simulink model "GNC"  (R2015b)
settings: Solver=ode45  StartTime=0.0  StopTime=15  MaxStep=0.1  RelTol=1e-3
InitFcn:
  | % load parameters of the default quadrotor
  | disp('Quadrotor parameters loaded by InitFcn')
  | mdl_quadrotor
undefined symbols (not defined in the file or in its folder): quad
libraries: roblocks x1, simulink x1
settings Model: Creator=corkep  LastModifiedBy=Borja
settings DataIOCC: SaveFormat=Array  SignalLoggingSaveFormat=ModelDataLogs
settings OptimizationCC: ExpressionDepthLimit=2147483647
settings DebuggingCC: UnderspecifiedInitializationDetection=Classic  MergeDetectMultiDrivingBlocksExec=none  SolverPrmCheckMsg=warning  FcnCallInpInsideContextMsg=UseLocalSettings  StateNameClashWarn=warning
settings HardwareCC: ProdBitPerPointer=32  ProdLargestAtomicFloat=None  ProdIntDivRoundTo=Undefined  ProdEndianess=Unspecified  ProdWordSize=32  ProdHWDeviceType=32-bit Generic
settings GRTTargetCC: GeneratePreprocessorConditionals=Disable all  CombineOutputUpdateFcns=off  GRTInterface=on
settings ConfigComp: CovModelRefEnable=Off  CovSFcnEnable=off

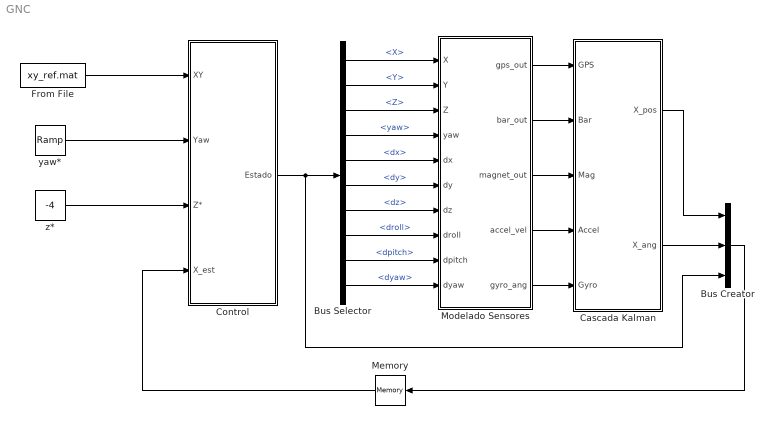
== system GNC ==
  Bus Creator : BusCreator  Inputs=3
  Bus Selector : BusSelector  OutputSignals=X,Y,Z,yaw,dx,dy,dz,droll,dpitch,dyaw
  Cascada Kalman : Subsystem
  Control : Subsystem
  From File : FromFile  FileName=xy_ref.mat  SampleTime=0
  Memory : Memory  InheritSampleTime=on
  Modelado Sensores : Subsystem
  yaw* : simulink/Sources/Ramp  slope=0.2  start=2  X0=0
  z* : Constant  Value=-4  SampleTime=0
  wires:
  Bus Selector/1 -> Modelado Sensores/1(X)  "<X>"
  Bus Selector/2 -> Modelado Sensores/2(Y)  "<Y>"
  Bus Selector/3 -> Modelado Sensores/3(Z)  "<Z>"
  Bus Selector/4 -> Modelado Sensores/4(yaw)  "<yaw>"
  Bus Selector/5 -> Modelado Sensores/5(dx)  "<dx>"
  Bus Selector/6 -> Modelado Sensores/6(dy)  "<dy>"
  Bus Selector/7 -> Modelado Sensores/7(dz)  "<dz>"
  Bus Selector/10 -> Modelado Sensores/10(dyaw)  "<dyaw>"
  Bus Selector/9 -> Modelado Sensores/9(dpitch)  "<dpitch>"
  Bus Selector/8 -> Modelado Sensores/8(droll)  "<droll>"
  Modelado Sensores/2(bar_out) -> Cascada Kalman/2(Bar)
  Modelado Sensores/3(magnet_out) -> Cascada Kalman/3(Mag)
  Modelado Sensores/4(accel_vel) -> Cascada Kalman/4(Accel)
  Modelado Sensores/5(gyro_ang) -> Cascada Kalman/5(Gyro)
  Control/1(Estado) -> Bus Creator/3, Bus Selector/1
  Cascada Kalman/1(X_pos) -> Bus Creator/1
  Bus Creator/1 -> Memory/1
  Cascada Kalman/2(X_ang) -> Bus Creator/2
  z*/1 -> Control/3(Z*)
  yaw*/1 -> Control/2(Yaw)
  Memory/1 -> Control/4(X_est)
  Modelado Sensores/1(gps_out) -> Cascada Kalman/1(GPS)
  From File/1 -> Control/1(XY)

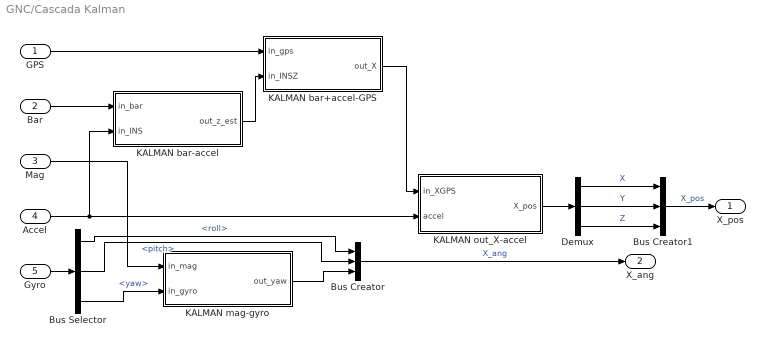
== system GNC/Cascada Kalman ==
  GPS : Inport
  Bar : Inport  Port=2
  Mag : Inport  Port=3
  Accel : Inport  Port=4
  Gyro : Inport  Port=5
  Bus Creator : BusCreator  Inputs=3
  Bus Creator1 : BusCreator  Inputs=3
  Bus Selector : BusSelector  OutputSignals=roll,pitch,yaw
  Demux : Demux  Outputs=3
  KALMAN bar+accel-GPS : Subsystem
  KALMAN bar-accel : Subsystem
  KALMAN mag-gyro : Subsystem
  KALMAN out_X-accel : Subsystem
  X_pos : Outport
  X_ang : Outport  Port=2
  wires:
  Accel/1 -> KALMAN out_X-accel/2(accel), KALMAN bar-accel/2(in_INS)
  GPS/1 -> KALMAN bar+accel-GPS/1(in_gps)
  KALMAN bar-accel/1(out_z_est) -> KALMAN bar+accel-GPS/2(in_INSZ)
  Bar/1 -> KALMAN bar-accel/1(in_bar)
  KALMAN bar+accel-GPS/1(out_X) -> KALMAN out_X-accel/1(in_XGPS)
  Gyro/1 -> Bus Selector/1
  Mag/1 -> KALMAN mag-gyro/1(in_mag)
  KALMAN mag-gyro/1(out_yaw) -> Bus Creator/3
  Bus Selector/2 -> Bus Creator/2  "<pitch>"
  Bus Selector/1 -> Bus Creator/1  "<roll>"
  Bus Selector/3 -> KALMAN mag-gyro/2(in_gyro)  "<yaw>"
  Bus Creator/1 -> X_ang/1  "X_ang"
  KALMAN out_X-accel/1(X_pos) -> Demux/1
  Demux/1 -> Bus Creator1/1  "X"
  Demux/2 -> Bus Creator1/2  "Y"
  Demux/3 -> Bus Creator1/3  "Z"
  Bus Creator1/1 -> X_pos/1  "X_pos"

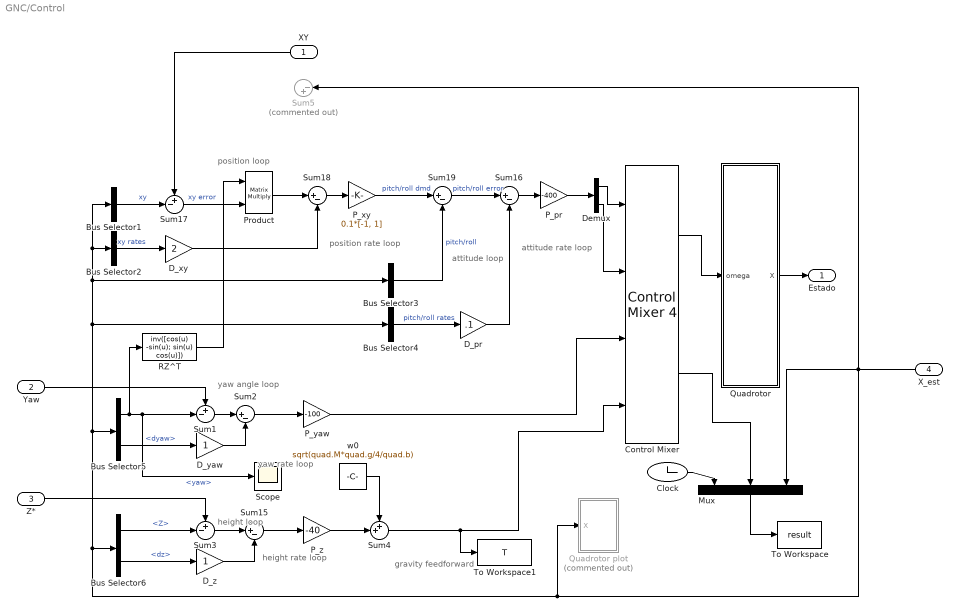
== system GNC/Control ==
  note: gravity feedforward
  note: attitude rate
      | loop
  note: attitude
      | loop
  note: position rate
      | loop
  note: position
      | loop
  note: yaw rate
      | loop
  note: yaw angle
      | loop
  note: height rate
      | loop
  note: height
      | loop
  XY : Inport
  Yaw : Inport  Port=2
  Z* : Inport  Port=3
  X_est : Inport  Port=4
  Bus Selector1 : BusSelector  OutputSignals=X_pos.X,X_pos.Y  OutputAsBus=on
  Bus Selector2 : BusSelector  OutputSignals=signal3.dx,signal3.dy  OutputAsBus=on
  Bus Selector3 : BusSelector  OutputSignals=X_ang.pitch,X_ang.roll  OutputAsBus=on
  Bus Selector4 : BusSelector  OutputSignals=signal3.dpitch,signal3.droll  OutputAsBus=on
  Bus Selector5 : BusSelector  OutputSignals=X_ang.yaw,signal3.dyaw
  Bus Selector6 : BusSelector  OutputSignals=X_pos.Z,signal3.dz
  Clock : Clock
  Control Mixer : roblocks/Dynamics/Control Mixer 4
  D_pr : Gain  Gain=.1
  D_xy : Gain  Gain=2
  D_yaw : Gain
  D_z : Gain
  Demux : Demux  Outputs=2
  Mux : Mux  Inputs=3
  P_pr : Gain  Gain=-400
  P_xy : Gain  Gain=0.1*[-1, 1]
  P_yaw : Gain  Gain=-100
  P_z : Gain  Gain=-40
  Product : Product  Multiplication=Matrix(*)  RndMeth=Zero
  Quadrotor : Subsystem  mask{quad=quad}
      mask prompts: quad "Quadrotor params"
      mask help: Quadrotor dynamics
      mask Help:
      | Integrate spatial velocity to update pose represented as a homogeneous
      | transformation.
      | 
      | <b>Parameters::</b>
      | 
      | q (struct)  A structure containing quadrotor dynamics
      | 
      | The elements of q are:
      | 
      |  J         Flyer rotational inertia matrix (3x3)
      |  h         Height of rotors above CoG (1x1)
      |  d         Length of flyer arms (1x1)
      |  nb        Number of blades per rotor (1x1)
      |  r         Rotor radius (1x1)
      |  c         Blade chord (1x1)
      |  e         Flapping hinge offset (1x1)
      |  Mb        Rotor blade mass (1x1)
      |  Mc        Estimated hub clamp mass (1x1)
      |  ec        Blade root clamp displacement (1x1)
      |  Ib        Rotor blade rotational inertia (1x1)
      |  Ic        Estimated root clamp inertia (1x1)
      |  mb        Static blade moment (1x1)
      |  Ir        Total rotor inertia (1x1)
      |  Ct        Non-dim. thrust coefficient (1x1)
      |  Cq        Non-dim. torque coefficient (1x1)
      |  sigma     Rotor solidity ratio (1x1)
      |  thetat    Blade tip angle (1x1)
      |  theta0    Blade root angle (1x1)
      |  theta1    Blade twist angle (1x1)
      |  theta75   3/4 blade angle (1x1)
      |  thetai    Blade ideal root approximation (1x1)
      |  a         Lift slope gradient (1x1)
      |  A         Rotor disc area (1x1)
      |  gamma     Lock number (1x1)
      | 
      | 
      | <b>Inputs::</b>
      | 
      | w1 (1x1) angular velocity of rotor 1 [rad]
      | w2 (1x1) angular velocity of rotor 2 [rad]
      | w3 (1x1) angular velocity of rotor 3 [rad]
      | w4 (1x1) angular velocity of rotor 4 [rad]
      | 
      | <b>Outputs::</b>
      | 
      | X (1x12) state vector (x, y, z, thr, thp, thy, xd, yd, zd, thrd, thpd, thyd)
      | 
      | (x,y,z) is the position in the world frame [m]
      | (thr, thp, thy) the roll/pitch/yaw orientation in the world frame [rad]
      | (xd,yd,zd) is the velocity in the body frame [m]
      | (thrd,thpd,thyd) is the roll/pitch/yaw rates in the body frame [rad/s]
      | 
      | <b>Notes::</b>
      | 
      | - See also mdl_quadrotor which defines parameters for the ANU X4 flyer.
  Quadrotor plot : Subsystem  Commented=on  mask{quad=quad, xydim=2, zdim=10}
      mask prompts: quad "Model"; xydim "xy-axes dimension"; zdim "z-axis dimension"
      mask help: Animate quadrotor.
      mask Help:
      | This block graphically displays a quadrotor (flying robot).
      | 
      | A new figure is created and A graphical model of a quadrotor is animated
      | to a pose specified by the state vector input to the block.
      | 
      | The state vector is [x y z roll pitch yaw] in world coordinates and the
      | angles are in radians.
      | 
      | Notes:
      | - The dimensions of the vehicle workspace are set by parameters
  RZ^T : MATLABFcn  MATLABFcn=inv([cos(u) -sin(u); sin(u) cos(u)])  OutputDimensions=[2 2]  Output1D=off
  Scope : Scope
  Sum1 : Sum  Inputs=+-|
  Sum{2,15..16,18..19} (5 alike) : Sum  Inputs=|+-
  Sum17 : Sum  Inputs=+-|
  Sum3 : Sum  Inputs=+-|
  Sum4 : Sum  Inputs=++|
  Sum5 : Sum  Commented=on  Inputs=|-+
  To Workspace : ToWorkspace  VariableName=result  SampleTime=-1
  To Workspace1 : ToWorkspace  VariableName=T  SampleTime=-1
  w0 : Constant  Value=sqrt(quad.M*quad.g/4/quad.b)  SampleTime=0
  Estado : Outport
  wires:
  w0/1 -> Sum4/1
  Sum15/1 -> P_z/1
  P_z/1 -> Sum4/2
  Quadrotor/1(X) -> Estado/1
  Bus Selector1/1 -> Sum17/2  "xy"
  Bus Selector2/1 -> D_xy/1  "xy rates"
  D_xy/1 -> Sum18/2
  P_xy/1 -> Sum19/1  "pitch/roll dmd"
  Bus Selector3/1 -> Sum19/2  "pitch/roll"
  Bus Selector4/1 -> D_pr/1  "pitch/roll rates"
  Sum19/1 -> Sum16/1  "pitch/roll error"
  Sum16/1 -> P_pr/1
  P_pr/1 -> Demux/1
  P_yaw/1 -> Control Mixer/3
  Bus Selector5/1 -> RZ^T/1, Sum1/2, Scope/1  "<yaw>"
  Sum2/1 -> P_yaw/1
  Z*/1 -> Sum3/1
  Bus Selector6/1 -> Sum3/2  "<Z>"
  Bus Selector5/2 -> D_yaw/1  "<dyaw>"
  Sum3/1 -> Sum15/1
  D_z/1 -> Sum15/2
  Bus Selector6/2 -> D_z/1  "<dz>"
  D_pr/1 -> Sum16/2
  Demux/2 -> Control Mixer/2
  D_yaw/1 -> Sum2/2
  Sum4/1 -> To Workspace1/1, Control Mixer/4
  Sum1/1 -> Sum2/1
  Mux/1 -> To Workspace/1
  Clock/1 -> Mux/1
  RZ^T/1 -> Product/1
  Sum18/1 -> P_xy/1
  Yaw/1 -> Sum1/1
  Product/1 -> Sum18/1
  Sum17/1 -> Product/2  "xy error"
  Demux/1 -> Control Mixer/1
  Control Mixer/1 -> Quadrotor/1(omega)
  X_est/1 -> Quadrotor plot/1(X), Bus Selector6/1, Bus Selector5/1, Bus Selector4/1, Bus Selector3/1, Bus Selector2/1, Bus Selector1/1, Sum5/1, Mux/3
  Control Mixer/2 -> Mux/2
  XY/1 -> Sum17/1

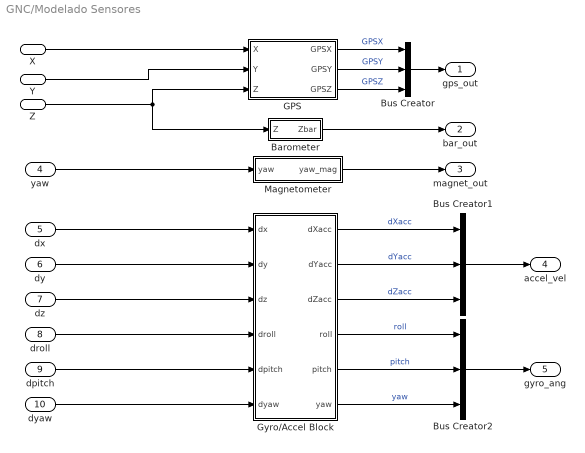
== system GNC/Modelado Sensores ==
  X : Inport
  Y : Inport  Port=2
  Z : Inport  Port=3
  yaw : Inport  Port=4
  dx : Inport  Port=5
  dy : Inport  Port=6
  dz : Inport  Port=7
  droll : Inport  Port=8
  dpitch : Inport  Port=9
  dyaw : Inport  Port=10
  Barometer : Subsystem
  Bus Creator : BusCreator  Inputs=3
  Bus Creator1 : BusCreator  Inputs='dXacc','dYacc','dZacc'
  Bus Creator2 : BusCreator  Inputs=3
  GPS : Subsystem
  Gyro/Accel Block : Subsystem
  Magnetometer : Subsystem
  gps_out : Outport
  bar_out : Outport  Port=2
  magnet_out : Outport  Port=3
  accel_vel : Outport  Port=4
  gyro_ang : Outport  Port=5
  wires:
  Bus Creator1/1 -> accel_vel/1
  Magnetometer/1(yaw_mag) -> magnet_out/1
  Bus Creator2/1 -> gyro_ang/1
  Barometer/1(Zbar) -> bar_out/1
  X/1 -> GPS/1(X)
  Y/1 -> GPS/2(Y)
  Z/1 -> GPS/3(Z), Barometer/1(Z)
  yaw/1 -> Magnetometer/1(yaw)
  GPS/1(GPSX) -> Bus Creator/1  "GPSX"
  GPS/2(GPSY) -> Bus Creator/2  "GPSY"
  GPS/3(GPSZ) -> Bus Creator/3  "GPSZ"
  Gyro/Accel Block/5(pitch) -> Bus Creator2/2  "pitch"
  Gyro/Accel Block/2(dYacc) -> Bus Creator1/2  "dYacc"
  Bus Creator/1 -> gps_out/1
  Gyro/Accel Block/1(dXacc) -> Bus Creator1/1  "dXacc"
  Gyro/Accel Block/3(dZacc) -> Bus Creator1/3  "dZacc"
  Gyro/Accel Block/6(yaw) -> Bus Creator2/3  "yaw"
  Gyro/Accel Block/4(roll) -> Bus Creator2/1  "roll"
  dx/1 -> Gyro/Accel Block/1(dx)
  dy/1 -> Gyro/Accel Block/2(dy)
  dz/1 -> Gyro/Accel Block/3(dz)
  dpitch/1 -> Gyro/Accel Block/5(dpitch)
  droll/1 -> Gyro/Accel Block/4(droll)
  dyaw/1 -> Gyro/Accel Block/6(dyaw)

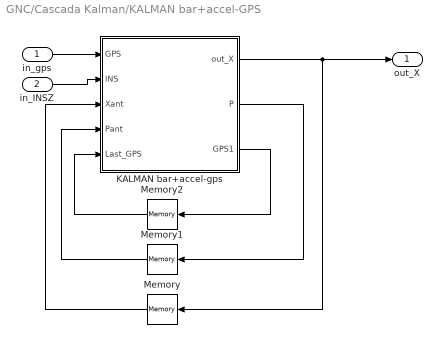
== system GNC/Cascada Kalman/KALMAN bar+accel-GPS ==
  in_gps : Inport
  in_INSZ : Inport  Port=2
  KALMAN bar+accel-gps : MATLAB Function  TreatAsAtomicUnit=on
  Memory : Memory  X0=[0;0;0]  InheritSampleTime=on
  Memory1 : Memory  X0=0.001  InheritSampleTime=on
  Memory2 : Memory  X0=0.001*[1;1;1]  InheritSampleTime=on
  out_X : Outport
  wires:
  in_gps/1 -> KALMAN bar+accel-gps/1(GPS)
  Memory/1 -> KALMAN bar+accel-gps/3(Xant)
  Memory1/1 -> KALMAN bar+accel-gps/4(Pant)
  KALMAN bar+accel-gps/3(GPS1) -> Memory2/1
  in_INSZ/1 -> KALMAN bar+accel-gps/2(INS)
  KALMAN bar+accel-gps/1(out_X) -> out_X/1, Memory/1
  KALMAN bar+accel-gps/2(P) -> Memory1/1
  Memory2/1 -> KALMAN bar+accel-gps/5(Last_GPS)

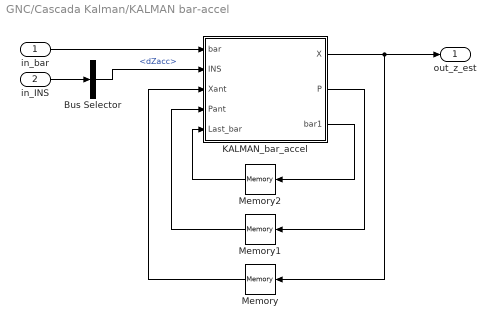
== system GNC/Cascada Kalman/KALMAN bar-accel ==
  in_bar : Inport
  in_INS : Inport  Port=2
  Bus Selector : BusSelector  OutputSignals=dZacc
  KALMAN_bar_accel : MATLAB Function  TreatAsAtomicUnit=on
  Memory : Memory
  Memory1 : Memory  X0=0.01  InheritSampleTime=on
  Memory2 : Memory  X0=0.001  InheritSampleTime=on
  out_z_est : Outport
  wires:
  in_bar/1 -> KALMAN_bar_accel/1(bar)
  KALMAN_bar_accel/1(X) -> Memory/1, out_z_est/1
  KALMAN_bar_accel/2(P) -> Memory1/1
  Memory1/1 -> KALMAN_bar_accel/4(Pant)
  Memory/1 -> KALMAN_bar_accel/3(Xant)
  KALMAN_bar_accel/3(bar1) -> Memory2/1
  Memory2/1 -> KALMAN_bar_accel/5(Last_bar)
  in_INS/1 -> Bus Selector/1
  Bus Selector/1 -> KALMAN_bar_accel/2(INS)  "<dZacc>"

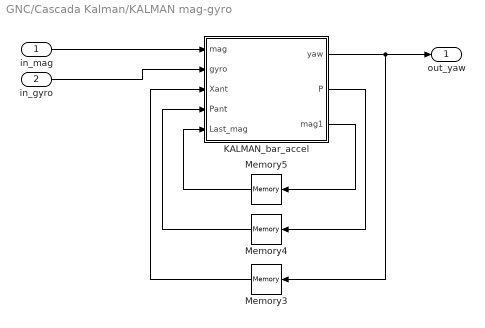
== system GNC/Cascada Kalman/KALMAN mag-gyro ==
  in_mag : Inport
  in_gyro : Inport  Port=2
  KALMAN_bar_accel : MATLAB Function  TreatAsAtomicUnit=on
  Memory3 : Memory  InheritSampleTime=on
  Memory4 : Memory  X0=0.01  InheritSampleTime=on
  Memory5 : Memory  X0=0.001  InheritSampleTime=on
  out_yaw : Outport
  wires:
  in_mag/1 -> KALMAN_bar_accel/1(mag)
  in_gyro/1 -> KALMAN_bar_accel/2(gyro)
  KALMAN_bar_accel/2(P) -> Memory4/1
  Memory4/1 -> KALMAN_bar_accel/4(Pant)
  Memory3/1 -> KALMAN_bar_accel/3(Xant)
  KALMAN_bar_accel/3(mag1) -> Memory5/1
  Memory5/1 -> KALMAN_bar_accel/5(Last_mag)
  KALMAN_bar_accel/1(yaw) -> out_yaw/1, Memory3/1

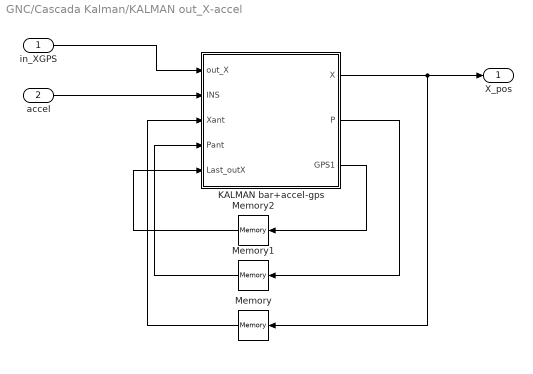
== system GNC/Cascada Kalman/KALMAN out_X-accel ==
  in_XGPS : Inport
  accel : Inport  Port=2
  KALMAN bar+accel-gps : MATLAB Function  TreatAsAtomicUnit=on
  Memory : Memory  X0=[-1;0;0]  InheritSampleTime=on
  Memory1 : Memory  X0=0.01*[1 0 0;0 1 0;0 0 1]  InheritSampleTime=on
  Memory2 : Memory  X0=0.001*[1;1;1]  InheritSampleTime=on
  X_pos : Outport
  wires:
  accel/1 -> KALMAN bar+accel-gps/2(INS)
  in_XGPS/1 -> KALMAN bar+accel-gps/1(out_X)
  Memory/1 -> KALMAN bar+accel-gps/3(Xant)
  Memory1/1 -> KALMAN bar+accel-gps/4(Pant)
  KALMAN bar+accel-gps/3(GPS1) -> Memory2/1
  KALMAN bar+accel-gps/1(X) -> Memory/1, X_pos/1
  KALMAN bar+accel-gps/2(P) -> Memory1/1
  Memory2/1 -> KALMAN bar+accel-gps/5(Last_outX)

== system GNC/Control/Quadrotor ==
  omega : Inport
  Bus Creator : BusCreator  Inputs='X','Y','Z','yaw','pitch','roll','dx','dy','dz','dyaw','dpitch','droll'
  Demux : Demux  Outputs=12
  Dynamics : S-Function  FunctionName=quadrotor_dynamics  Parameters=quad  SFunctionDeploymentMode=off  EnableBusSupport=off
  X : Outport
  wires:
  Demux/1 -> Bus Creator/1  "X"
  Demux/3 -> Bus Creator/3  "Z"
  Demux/4 -> Bus Creator/4  "yaw"
  Demux/5 -> Bus Creator/5  "pitch"
  omega/1 -> Dynamics/1
  Demux/7 -> Bus Creator/7  "dx"
  Demux/9 -> Bus Creator/9  "dz"
  Demux/2 -> Bus Creator/2  "Y"
  Demux/6 -> Bus Creator/6  "roll"
  Demux/8 -> Bus Creator/8  "dy"
  Bus Creator/1 -> X/1
  Dynamics/1 -> Demux/1
  Demux/10 -> Bus Creator/10  "dyaw"
  Demux/11 -> Bus Creator/11  "dpitch"
  Demux/12 -> Bus Creator/12  "droll"

== system GNC/Control/Quadrotor plot ==
  X : Inport
  Bus Selector1 : BusSelector  OutputSignals=X_pos.X,X_pos.Y,X_pos.Z,X_ang.roll,X_ang.pitch,X_ang.yaw  OutputAsBus=on
  Plotter : S-Function  FunctionName=quadrotor_plot  Parameters=[xydim, zdim], 1, 1,quad  SFunctionDeploymentMode=off  EnableBusSupport=off
  wires:
  X/1 -> Bus Selector1/1
  Bus Selector1/1 -> Plotter/1

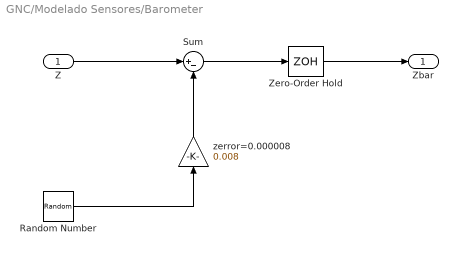
== system GNC/Modelado Sensores/Barometer ==
  Z : Inport
  Random Number : RandomNumber  SampleTime=0.1
  Sum : Sum  Inputs=|+-
  Zero-Order Hold : ZeroOrderHold  SampleTime=1/10
  zerror=0.000008 : Gain  Gain=0.008
  Zbar : Outport
  wires:
  Z/1 -> Sum/1
  zerror=0.000008/1 -> Sum/2
  Random Number/1 -> zerror=0.000008/1
  Sum/1 -> Zero-Order Hold/1
  Zero-Order Hold/1 -> Zbar/1

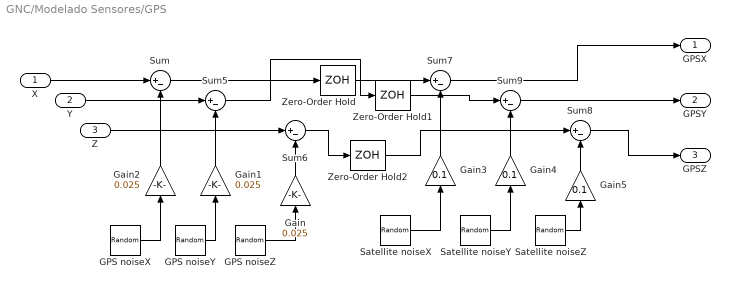
== system GNC/Modelado Sensores/GPS ==
  X : Inport
  Y : Inport  Port=2
  Z : Inport  Port=3
  GPS noiseX : RandomNumber  SampleTime=0.1
  GPS noiseY : RandomNumber  SampleTime=0.1
  GPS noiseZ : RandomNumber  SampleTime=0.1
  Gain : Gain  Gain=0.025
  Gain1 : Gain  Gain=0.025
  Gain2 : Gain  Gain=0.025
  Gain3 : Gain  Gain=0.1
  Gain4 : Gain  Gain=0.1
  Gain5 : Gain  Gain=0.1
  Satellite noiseX : RandomNumber  SampleTime=2
  Satellite noiseY : RandomNumber  SampleTime=2
  Satellite noiseZ : RandomNumber  SampleTime=2
  Sum{,5..9} (6 alike) : Sum  Inputs=|+-
  Zero-Order Hold : ZeroOrderHold  SampleTime=1/10
  Zero-Order Hold1 : ZeroOrderHold  SampleTime=1/10
  Zero-Order Hold2 : ZeroOrderHold  SampleTime=1/10
  GPSX : Outport
  GPSY : Outport  Port=2
  GPSZ : Outport  Port=3
  wires:
  GPS noiseY/1 -> Gain1/1
  GPS noiseZ/1 -> Gain/1
  GPS noiseX/1 -> Gain2/1
  Satellite noiseZ/1 -> Gain5/1
  Satellite noiseX/1 -> Gain3/1
  Satellite noiseY/1 -> Gain4/1
  Sum9/1 -> GPSY/1
  Sum8/1 -> GPSZ/1
  Gain3/1 -> Sum7/2
  Gain/1 -> Sum6/2
  Gain1/1 -> Sum5/2
  Gain2/1 -> Sum/2
  Gain5/1 -> Sum8/2
  Sum7/1 -> GPSX/1
  Gain4/1 -> Sum9/2
  Z/1 -> Sum6/1
  X/1 -> Sum/1
  Y/1 -> Sum5/1
  Sum/1 -> Zero-Order Hold/1
  Zero-Order Hold/1 -> Sum7/1
  Sum5/1 -> Zero-Order Hold1/1
  Zero-Order Hold1/1 -> Sum9/1
  Sum6/1 -> Zero-Order Hold2/1
  Zero-Order Hold2/1 -> Sum8/1

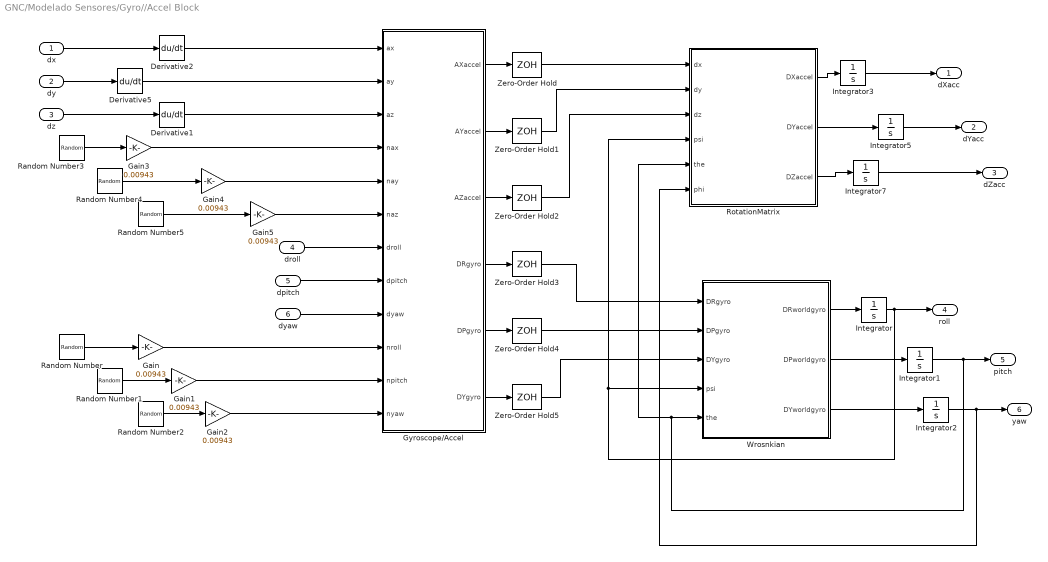
== system GNC/Modelado Sensores/Gyro//Accel Block ==
  dx : Inport
  dy : Inport  Port=2
  dz : Inport  Port=3
  droll : Inport  Port=4
  dpitch : Inport  Port=5
  dyaw : Inport  Port=6
  Derivative1 : Derivative
  Derivative2 : Derivative
  Derivative5 : Derivative
  Gain{,1..5} (6 alike) : Gain  Gain=0.00943
  Gyroscope/Accel : MATLAB Function  TreatAsAtomicUnit=on
  Integrator{,1..3,5,7} (6 alike) : Integrator
  Random Number{,1..5} (6 alike) : RandomNumber  Variance=0.00943  SampleTime=1/330
  RotationMatrix : MATLAB Function  TreatAsAtomicUnit=on
  Wrosnkian : MATLAB Function  TreatAsAtomicUnit=on
  Zero-Order Hold{,1..5} (6 alike) : ZeroOrderHold  SampleTime=1/330
  dXacc : Outport
  dYacc : Outport  Port=2
  dZacc : Outport  Port=3
  roll : Outport  Port=4
  pitch : Outport  Port=5
  yaw : Outport  Port=6
  wires:
  dyaw/1 -> Gyroscope/Accel/9(dyaw)
  dpitch/1 -> Gyroscope/Accel/8(dpitch)
  droll/1 -> Gyroscope/Accel/7(droll)
  Gyroscope/Accel/6(DYgyro) -> Zero-Order Hold5/1
  Random Number/1 -> Gain/1
  Gain1/1 -> Gyroscope/Accel/11(npitch)
  Random Number1/1 -> Gain1/1
  Random Number2/1 -> Gain2/1
  Gain2/1 -> Gyroscope/Accel/12(nyaw)
  Gain/1 -> Gyroscope/Accel/10(nroll)
  Gain4/1 -> Gyroscope/Accel/5(nay)
  Random Number4/1 -> Gain4/1
  Random Number5/1 -> Gain5/1
  Gain5/1 -> Gyroscope/Accel/6(naz)
  Random Number3/1 -> Gain3/1
  Gain3/1 -> Gyroscope/Accel/4(nax)
  Gyroscope/Accel/1(AXaccel) -> Zero-Order Hold/1
  Integrator3/1 -> dXacc/1
  Gyroscope/Accel/2(AYaccel) -> Zero-Order Hold1/1
  Gyroscope/Accel/3(AZaccel) -> Zero-Order Hold2/1
  dx/1 -> Derivative2/1
  dy/1 -> Derivative5/1
  dz/1 -> Derivative1/1
  Derivative2/1 -> Gyroscope/Accel/1(ax)
  Derivative5/1 -> Gyroscope/Accel/2(ay)
  Derivative1/1 -> Gyroscope/Accel/3(az)
  Gyroscope/Accel/4(DRgyro) -> Zero-Order Hold3/1
  Gyroscope/Accel/5(DPgyro) -> Zero-Order Hold4/1
  Zero-Order Hold/1 -> RotationMatrix/1(dx)
  Zero-Order Hold1/1 -> RotationMatrix/2(dy)
  Zero-Order Hold2/1 -> RotationMatrix/3(dz)
  RotationMatrix/1(DXaccel) -> Integrator3/1
  RotationMatrix/2(DYaccel) -> Integrator5/1
  RotationMatrix/3(DZaccel) -> Integrator7/1
  Zero-Order Hold3/1 -> Wrosnkian/1(DRgyro)
  Zero-Order Hold4/1 -> Wrosnkian/2(DPgyro)
  Zero-Order Hold5/1 -> Wrosnkian/3(DYgyro)
  Wrosnkian/1(DRworldgyro) -> Integrator/1
  Wrosnkian/2(DPworldgyro) -> Integrator1/1
  Wrosnkian/3(DYworldgyro) -> Integrator2/1
  Integrator/1 -> roll/1, RotationMatrix/4(psi), Wrosnkian/4(psi)
  Integrator1/1 -> RotationMatrix/5(the), Wrosnkian/5(the), pitch/1
  Integrator2/1 -> RotationMatrix/6(phi), yaw/1
  Integrator5/1 -> dYacc/1
  Integrator7/1 -> dZacc/1

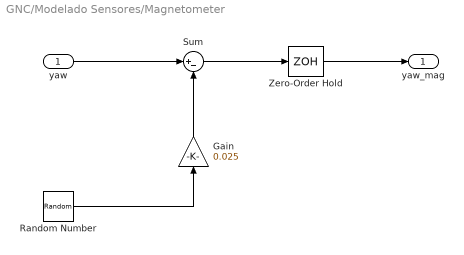
== system GNC/Modelado Sensores/Magnetometer ==
  yaw : Inport
  Gain : Gain  Gain=0.025
  Random Number : RandomNumber  SampleTime=0.1
  Sum : Sum  Inputs=|+-
  Zero-Order Hold : ZeroOrderHold  SampleTime=1/10
  yaw_mag : Outport
  wires:
  yaw/1 -> Sum/1
  Gain/1 -> Sum/2
  Random Number/1 -> Gain/1
  Sum/1 -> Zero-Order Hold/1
  Zero-Order Hold/1 -> yaw_mag/1

== matlab function GNC/Cascada Kalman/KALMAN bar+accel-GPS/KALMAN bar+accel-gps ==
  data: GPS input; out_X output; INS input; Xant input; P output; Pant input; GPS1 output; Last_GPS input
function [out_X,P,GPS1] = kalman(GPS,INS,Xant,Pant,Last_GPS)
% FILTRO DE KALMAN ACELEROMETRO - GPS
R = 0.001;
H = 1;
Q = 0.001;
% PREDICCION DEL ESTADO 
% 1) Estimacion de la posicion con los datos de acelerometro
X = INS;
% 2) Estimacion de la matriz P
A = 1;
B = INS;
P = A*Pant*A' + Q;
% INNOVACION EN LA MEDIDA Y CORRECCION, SI CORRESPONDE
% 3) Medida estimada Z_est y medida del GPS, Z
Z_est = H*X;
Z = GPS(3);
if isequal(GPS(3),Last_GPS(3)) == 0,
    Y = Z-Z_est;
    S = H*P*H' + R;
    K = P*H'*inv(S);
    X = X + K*Y;
    P = (1-K*H)*P;
else
    % do nothing
end
GPS1 = GPS;
out_X = [GPS(1);GPS(2);X];

== matlab function GNC/Cascada Kalman/KALMAN bar-accel/KALMAN_bar_accel ==
  data: bar input; X output; INS input; Xant input; P output; Pant input; bar1 output; Last_bar input
function [X,P,bar1] = kalman(bar,INS,Xant,Pant,Last_bar)
% FILTRO DE KALMAN ACELEROMETRO - GPS
R = 0.001;
H = 1;
Q = 0.001;
% INS = INS(3);   % Solo la componente en altura Z
% PREDICCION DEL ESTADO 
% 1) Estimacion de la posicion con los datos de acelerometro
X = Xant + 0.0030303*INS;
% 2) Estimacion de la matriz P
A = 1;
% B = INS;
P = A*Pant*A' + Q;
% INNOVACION EN LA MEDIDA Y CORRECCION, SI CORRESPONDE
% 3) Medida estimada Z_est y medida del GPS, Z
Z_est = H*X;
Z = bar;
if isequal(bar,Last_bar) == 0,
    Y = Z-Z_est;
    S = H*P*H' + R;
    K = P*H'*inv(S);
    X = X + K*Y;
    P = (1-K*H)*P;
else
    % do nothing
end
bar1 = bar;

== matlab function GNC/Cascada Kalman/KALMAN out_X-accel/KALMAN bar+accel-gps ==
  data: out_X input; X output; INS input; Xant input; P output; Pant input; GPS1 output; Last_outX input
function [X,P,GPS1] = kalman(out_X,INS,Xant,Pant,Last_outX)
% FILTRO DE KALMAN ACELEROMETRO - GPS
R = 0.001*eye(3);
H = eye(3);
Q = 0.001*eye(3);
% PREDICCION DEL ESTADO 
% 1) Estimacion de la posicion con los datos de acelerometro
X = Xant + 0.0030303*INS;
% 2) Estimacion de la matriz P
A = eye(3);
P = A*Pant*A' + Q;
% INNOVACION EN LA MEDIDA Y CORRECCION, SI CORRESPONDE
% 3) Medida estimada Z_est y medida del GPS, Z
Z_est = H*X;
Z = out_X;
if isequal(out_X,Last_outX) == 0,
    Y = Z-Z_est;
    S = H*P*H' + R;
    K = P*H'*inv(S);
    X = X + K*Y;
    P = (eye(3)-K*H)*P;
else
    % do nothing
end
GPS1 = out_X;

== matlab function GNC/Cascada Kalman/KALMAN mag-gyro/KALMAN_bar_accel ==
  data: mag input; yaw output; gyro input; Xant input; P output; Pant input; mag1 output; Last_mag input
function [yaw,P,mag1] = kalman(mag,gyro,Xant,Pant,Last_mag)
% FILTRO DE KALMAN ACELEROMETRO - GPS
R = 0.001;
H = 1;
Q = 0.001;
% PREDICCION DEL ESTADO 
% 1) Estimacion de la posicion con los datos de acelerometro
yaw = Xant + 0.0030303*gyro;
% 2) Estimacion de la matriz P
A = 1;
B = gyro;
P = A*Pant*A' + Q;
% INNOVACION EN LA MEDIDA Y CORRECCION, SI CORRESPONDE
% 3) Medida estimada Z_est y medida del GPS, Z
Z_est = H*yaw;
Z = mag;
if isequal(mag,Last_mag) == 0,
    Y = Z-Z_est;
    S = H*P*H' + R;
    K = P*H'*inv(S);
    yaw = yaw + K*Y;
    P = (1-K*H)*P;
else
    % do nothing
end
mag1 = mag;

== matlab function GNC/Modelado Sensores/Gyro//Accel Block/Gyroscope//Accel ==
  data: AXaccel output; AYaccel output; AZaccel output; ax input; ay input; az input; nax input; nay input; naz input; DRgyro output; DPgyro output; DYgyro output; droll input; dpitch input; dyaw input; nroll input; npitch input; nyaw input
function [AXaccel,AYaccel,AZaccel,DRgyro,DPgyro,DYgyro] = fcn(ax,ay,az,nax,nay,naz,droll,dpitch,dyaw,nroll,npitch,nyaw)
%%Valores Gyroscopo
%Sx: Sensibilidad. Bf: Ruido de salida. Mxyz:Misalignment
Sxgyro = 0.000175;
Bfgyro = 0.00047;
Mxgyro = 0.00175;
Mygyro = 0.00175;
Mzgyro = 0.00175;
%%Valores Accel
Sxacc = 0.000833;
Bfacc = 0.00051;
%Misalignment 0.2º = 0.004g
Mxacc = 0.004;
Myacc = 0.004;
Mzacc = 0.004;
%Droll dpitch dyaw to axis (from Body Frame to World)
DRPY = [dyaw;dpitch;droll];
%Acceleration from body frame to World
AXYZ = [ax;ay;az];
%Apply the Accel Model
AXaccel = (1+Sxacc)*AXYZ(1)+Myacc*AXYZ(2)+Mzacc*AXYZ(3)+Bfacc+nax;
AYaccel = (1+Sxacc)*AXYZ(2)+Mxacc*AXYZ(1)+Mzacc*AXYZ(3)+Bfacc+nay;
AZaccel = (1+Sxacc)*AXYZ(3)+Mxacc*AXYZ(1)+Myacc*AXYZ(2)+Bfacc+naz;
%Apply the Gyro Model
DRgyro = (1+Sxgyro)*DRPY(1)+Mygyro*DRPY(2)+Mzgyro*DRPY(3)+Bfgyro+nroll;
DPgyro = (1+Sxgyro)*DRPY(2)+Mxgyro*DRPY(1)+Mzgyro*DRPY(3)+Bfgyro+npitch;
DYgyro = (1+Sxgyro)*DRPY(3)+Mxgyro*DRPY(1)+Mygyro*DRPY(2)+Bfgyro+nyaw;

== matlab function GNC/Modelado Sensores/Gyro//Accel Block/RotationMatrix ==
  data: DXaccel output; DYaccel output; DZaccel output; dx input; dy input; dz input; psi input; the input; phi input
function [DXaccel,DYaccel,DZaccel] = fcn(dx,dy,dz,psi,the,phi)

%Rotation Matrix [rotz(phi)*roty(the)*rotx(psi)]
R = [cos(the)*cos(phi) sin(psi)*sin(the)*cos(phi)-cos(psi)*sin(phi) cos(psi)*sin(the)*cos(phi)+sin(psi)*sin(phi);   %BBF > Inertial rotation matrix
     cos(the)*sin(phi) sin(psi)*sin(the)*sin(phi)+cos(psi)*cos(phi) cos(psi)*sin(the)*sin(phi)-sin(psi)*cos(phi);
     -sin(the)         sin(psi)*cos(the)                            cos(psi)*cos(the)];
%Acceleration from body frame to World
DXYZ = R*[dx;dy;dz];

DXaccel = DXYZ(1);
DYaccel = DXYZ(2);
DZaccel = DXYZ(3);

== matlab function GNC/Modelado Sensores/Gyro//Accel Block/Wrosnkian ==
  data: DRworldgyro output; DPworldgyro output; DYworldgyro output; DRgyro input; DPgyro input; DYgyro input; psi input; the input
function [DRworldgyro,DPworldgyro,DYworldgyro] = fcn(DRgyro,DPgyro,DYgyro,psi,the)

%inverted Wronskian
iW = [0        sin(psi)          cos(psi);           
    0        cos(psi)*cos(the) -sin(psi)*cos(the);
    cos(the) sin(psi)*sin(the) cos(psi)*sin(the)] / cos(the);
%Acceleration from body frame to World
DRPY = inv(iW)*[DRgyro;DPgyro;DYgyro];
DRworldgyro = DRPY(1);
DPworldgyro = DRPY(2);
DYworldgyro = DRPY(3);
